simulink model "SmartRobotCar"  (R2026a)
settings: Solver=FixedStepDiscrete  StopTime=inf  FixedStep=0.01  EnableMultiTasking=on
libraries: arduinolib x1, arduinosensorlib x1
settings Model: SILPILModeSetting=veronly  ExtModeTrigDuration=2  Creator=cytech  LastModifiedBy=cytech
settings HardwareCC: ProdLargestAtomicInteger=Long  ProdLargestAtomicFloat=Double  ProdHWDeviceType=ARM Compatible->ARM Cortex  UseEmbeddedCoderFeatures=off  UseSimulinkCoderFeatures=off
settings RTWCC: SystemTargetFile=ert.tlc  HardwareBoard=ESP32-WROOM (Arduino Compatible)  TLCOptions="-aInlineSetEventsForThisBaseRateFcn=TLC_FALSE -aSuppressMultiTaskScheduler=TLC_FALSE  -aRateBasedStepFcn=0"  Toolchain=ESP32  BuildConfiguration=Faster Runs  Description=Embedded Coder
settings ERTTargetCC: ExtModeTransport=3.0  ExtModeAutomaticAllocSize=off  ExtModeStaticAllocSize=65536.0  SupportContinuousTime=on  SupportNonInlinedSFcns=on  SupportVariableSizeSignals=on

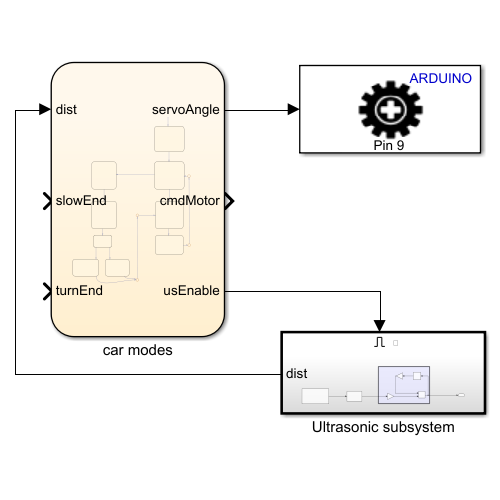
[thumbnail: Simulink's stored preview of the top-level diagram]
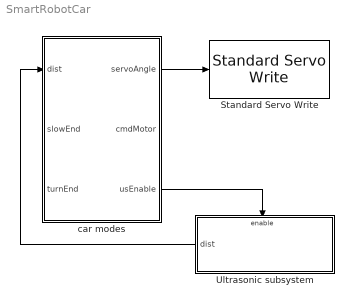
== system SmartRobotCar ==
  Standard Servo Write : arduinolib/Standard Servo Write  pinNumber=9  ServoIndex=0  blockPlatform=ARDUINO
  Ultrasonic subsystem : Subsystem
  car modes : Stateflow chart  TreatAsAtomicUnit=on
  wires:
  car modes/1(servoAngle) -> Standard Servo Write/1
  car modes/3(usEnable) -> Ultrasonic subsystem/Enable
  Ultrasonic subsystem/1(dist) -> car modes/1(dist)

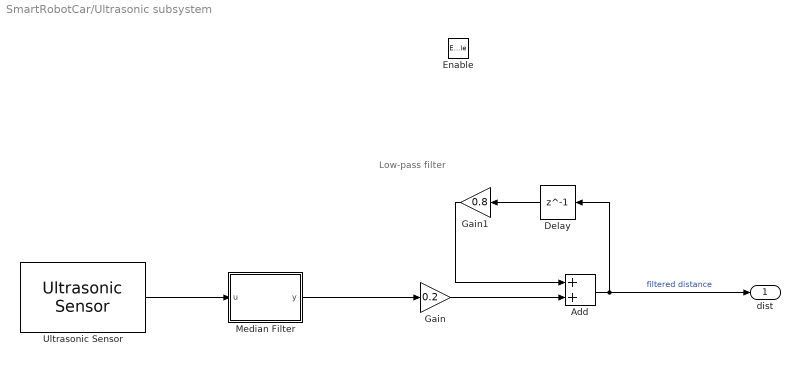
== system SmartRobotCar/Ultrasonic subsystem ==
  note: Low-pass filter
  Enable : EnablePort
  Add : Sum
  Delay : Delay  DelayLength=1
  Gain : Gain  Gain=0.2
  Gain1 : Gain  Gain=0.8
  Median Filter : MATLAB Function  TreatAsAtomicUnit=on
  Ultrasonic Sensor : arduinosensorlib/Ultrasonic Sensor  NumSignalPins=2  TrigPin=4  EchoPin=5  SignalPin=3  SampleTime_=0.1  blockPlatform=ARDUINO
  dist : Outport
  wires:
  Add/1 -> Delay/1, dist/1  "filtered distance"
  Ultrasonic Sensor/1 -> Median Filter/1(u)
  Gain/1 -> Add/2
  Delay/1 -> Gain1/1
  Gain1/1 -> Add/1
  Median Filter/1(y) -> Gain/1

== matlab function SmartRobotCar/Ultrasonic subsystem/Median Filter ==
  data: u input; y output
function y = medianFilter(u)
    % u est la mesure actuelle du capteur
    % On garde en mémoire les 3 dernières mesures
    persistent buffer
    if isempty(buffer)
        buffer = [u; u; u]; % Initialisation
    end
    
    % On décale le buffer et on ajoute la nouvelle valeur
    buffer = [buffer(2:end); u];
    
    % On prend la valeur du milieu (la médiane)
    y = median(buffer);
end

== stateflow chart SmartRobotCar/car modes ==
  state Initialisation
    entry:
    servoAngle=90
    cmdMotor=0
    usEnable=0
  state Check_left
    entry:
    servoAngle=135
    cmdMotor=0
    exit:
    distLeft=dist
  state Check_front
    entry:
    cmdMotor=0
    usEnable=1
    servoAngle=90
    exit:
    dist_front = dist
  state Move_forward
    entry:
    cmdMotor=1
    servoAngle=90
  state Check_right
    entry:
    servoAngle=45
    cmdMotor=0
    exit:
    distRight=dist
  state Decision
  state Slowdown
    entry:
    cmdMotor=5
  state turnLeft
    entry:
    cmdMotor=3
    servoAngle=90
  state turnRight
    entry:
    cmdMotor=2
    servoAngle=90
  (default) -> Initialisation
  Initialisation -> Check_front : after(0.5, sec)
  Check_front -> Check_left [order 2] : after(0,4, sec) [dist < 60]
  (junction 57) -> Check_front
  (junction 55) -> (junction 57) : [slowEnd == 1]
  Check_left -> Check_right : after(0,4, sec)
  Check_front -> Move_forward [order 1] : after(0,4, sec) [dist >= 60]
  (junction 51) -> Move_forward
  (junction 39) -> (junction 51) : [turnEnd ==1 ]
  Move_forward -> Slowdown : [dist < 40]
  Check_right -> Decision
  Slowdown -> (junction 55)
  Decision -> turnLeft [order 2] : [distLeft >= distRight]
  Decision -> turnRight [order 1] : [distRight > distLeft]
  turnRight -> (junction 39)
  turnLeft -> (junction 39)
  data: servoAngle output; cmdMotor output; usEnable output; dist input; dist_front local; distLeft local; distRight local; slowEnd input; turnEnd input
